simulink model "hilbert_example"  (R2024a)
settings: Solver=VariableStepAuto  StartTime=0.0  StopTime=10.0  RelTol=1e-3
model workspace (MAT data in the model file):
  ADC_BIT_RESOLUTION = 8
  ADC_BUFFER_SIZE = 1024
  ADC_Q_INTERVAL = 1
undefined symbols (not defined in the file): fdesignblkfcn, gcbh
libraries: dspxfrm3 x2
settings Model: Creator=94410  LastModifiedBy=94410

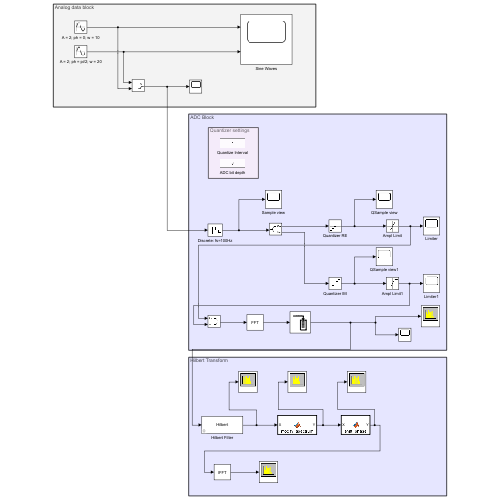
[thumbnail: Simulink's stored preview of the top-level diagram]
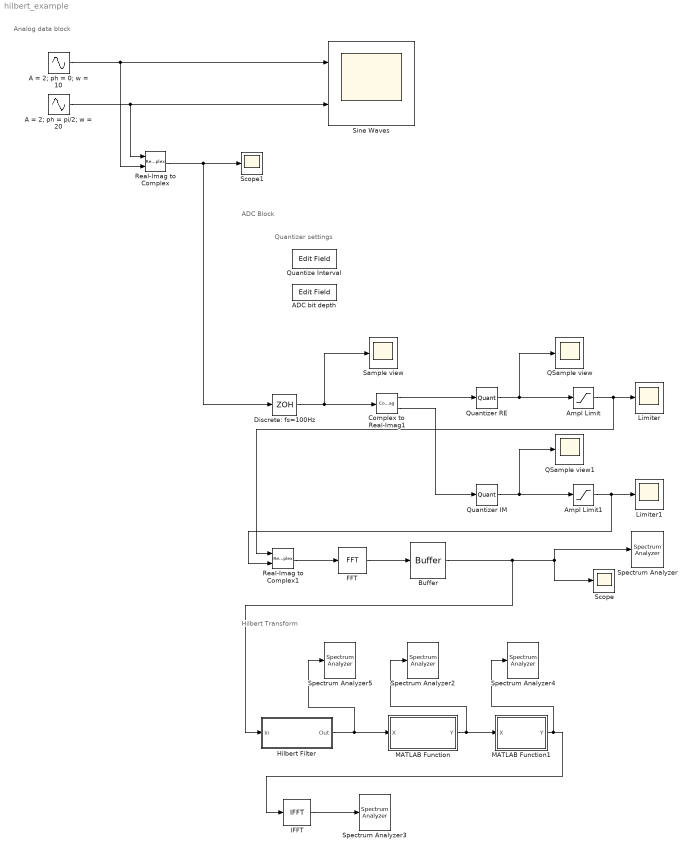
== system hilbert_example ==
  note: Hilbert Transform
  note: Quantizer settings
  note: Analog data block
  note: ADC Block
  A = 2; ph = 0; w = 10 : Sin  Amplitude=2  Frequency=10  SampleTime=0
  A = 2; ph = pi/2; w = 20 : Sin  Amplitude=2  Frequency=20  Phase=pi/2  SampleTime=0
  ADC bit depth : EditField  LabelPosition=Hide  ShowInitialText=on  Alignment=Center
  Ampl Limit : Saturate  UpperLimit=5  LowerLimit=-5
  Ampl Limit1 : Saturate  UpperLimit=5  LowerLimit=-5
  Buffer : Buffer  OutputFrames=off
  Complex to Real-Imag1 : ComplexToRealImag
  Discrete: fs=100Hz : ZeroOrderHold  SampleTime=0.01
  FFT : dspxfrm3/FFT  FFTImplementation=Auto  CompMethod=Table lookup  TableOpt=NEW  TableOptActive=Speed  BitRevOrder=off  Normalize=off  InheritFFTLength=on  FFTLength=64  WrapInput=on  roundingMode=Ceiling  overflowMode=off  firstCoeffDataTypeStr=Inherit: Same word length as input  firstCoeffLastDataTypeStr=Inherit: Same word length as input  outputMin=[]  outputMax=[]
  Hilbert Filter : Subsystem  DialogController=fdesignblkfcn  InitFcn=fdesignblkfcn(gcbh, {'InitFcn'});  mask(Hilbert Filter){}
      mask help: dsp:DSPFilterDesignBlockDialog:HilbertFdesign_MaskDesc
      settings: CopyFcn=fdesignblkfcn(gcbh, {'CopyFcn'});
      mask Help: helpview(mapfilelocation('dsp'), 'dsphilbertfilter');
      mask Display: disp('Hilbert')
  IFFT : dspxfrm3/IFFT  FFTImplementation=Auto  CompMethod=Table lookup  TableOpt=NEW  TableOptActive=Speed  BitRevOrder=off  cs_in=off  Normalize=on  InheritFFTLength=on  FFTLength=64  WrapInput=on  mode=Real  outSamplingMode=Sample based  roundingMode=Ceiling  overflowMode=off  firstCoeffDataTypeStr=Inherit: Same word length as input  firstCoeffLastDataTypeStr=Inherit: Same word length as input  outputMin=[]  outputMax=[]
  Limiter : Scope
  Limiter1 : Scope
  MATLAB Function : MATLAB Function  TreatAsAtomicUnit=on
  MATLAB Function1 : MATLAB Function  TreatAsAtomicUnit=on
  QSample view : Scope
  QSample view1 : Scope
  Quantize Interval : EditField  LabelPosition=Hide  ShowInitialText=on  Alignment=Center
  Quantizer IM : Quantizer  QuantizationInterval=ADC_Q_INTERVAL/(2^ADC_BIT_RESOLUTION)  LinearizeAsGain=off
  Quantizer RE : Quantizer  QuantizationInterval=ADC_Q_INTERVAL/(2^ADC_BIT_RESOLUTION)  LinearizeAsGain=off
  Real-Imag to Complex : RealImagToComplex
  Real-Imag to Complex1 : RealImagToComplex
  Sample view : Scope
  Scope : Scope
  Scope1 : Scope
  Sine Waves : Scope  NumInputPorts=2
  Spectrum Analyzer : SpectrumAnalyzer  WindowPosition=[355.000000,-231.000000,1318.000000,670.000000,]  ScopeFrameLocation=window  InputDomain=Frequency  Span=100  StartFrequency=-50  StopFrequency=50  InputUnits=None  SpectrumUnits=Auto  YLimits=[-2.5,2.5]  SelectedToolstripTab=spectrumAnalyzerToolstrip.channelMeasurementsTab
  Spectrum Analyzer2 : SpectrumAnalyzer  WindowPosition=[306.000000,180.000000,789.000000,436.000000,]  ScopeFrameLocation=window  InputDomain=Frequency  Span=100  StartFrequency=-50  StopFrequency=50  InputUnits=None  SpectrumUnits=Auto  YLimits=[-3.73353184,2.69746606]  SelectedToolstripTab=spectrumAnalyzerToolstrip.measurementsTab
  Spectrum Analyzer3 : SpectrumAnalyzer  WindowPosition=[266.000000,181.000000,1327.000000,750.000000,]  ScopeFrameLocation=window  InputDomain=Frequency  Span=100  StartFrequency=-50  StopFrequency=50  InputUnits=None  SpectrumUnits=Auto  YLimits=[-72.37843593,8.44661924]  SelectedToolstripTab=spectrumAnalyzerToolstrip.estimationTab
  Spectrum Analyzer4 : SpectrumAnalyzer  WindowPosition=[148.000000,72.000000,1242.000000,717.000000,]  ScopeFrameLocation=window  InputDomain=Frequency  Span=100  StartFrequency=-50  StopFrequency=50  InputUnits=None  SpectrumUnits=Auto  YLimits=[-1.91256104,2.64464345]
  Spectrum Analyzer5 : SpectrumAnalyzer  WindowPosition=[436.000000,73.000000,1242.000000,717.000000,]  ScopeFrameLocation=window  InputDomain=Frequency  Span=100  StartFrequency=-50  StopFrequency=50  InputUnits=None  SpectrumUnits=Auto  YLimits=[-61.42039238,37.54707884]  SelectedToolstripTab=spectrumAnalyzerToolstrip.measurementsTab
  wires:
  A = 2; ph = pi/2; w = 20/1 -> Real-Imag to Complex/1, Sine Waves/2
  A = 2; ph = 0; w = 10/1 -> Real-Imag to Complex/2, Sine Waves/1
  Quantizer RE/1 -> Ampl Limit/1, QSample view/1
  Ampl Limit/1 -> Real-Imag to Complex1/1, Limiter/1
  Real-Imag to Complex/1 -> Scope1/1, Discrete: fs=100Hz/1
  Discrete: fs=100Hz/1 -> Complex to Real-Imag1/1, Sample view/1
  Complex to Real-Imag1/1 -> Quantizer RE/1
  Ampl Limit1/1 -> Real-Imag to Complex1/2, Limiter1/1
  Quantizer IM/1 -> Ampl Limit1/1, QSample view1/1
  Complex to Real-Imag1/2 -> Quantizer IM/1
  Real-Imag to Complex1/1 -> FFT/1
  FFT/1 -> Buffer/1
  Buffer/1 -> Hilbert Filter/1(In), Spectrum Analyzer/1, Scope/1
  Hilbert Filter/1(Out) -> Spectrum Analyzer5/1, MATLAB Function/1(X)
  MATLAB Function/1(Y) -> Spectrum Analyzer2/1, MATLAB Function1/1(X)
  MATLAB Function1/1(Y) -> Spectrum Analyzer4/1, IFFT/1
  IFFT/1 -> Spectrum Analyzer3/1

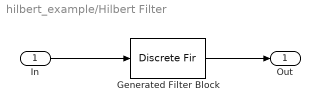
== system hilbert_example/Hilbert Filter ==
  In : Inport
  Generated Filter Block : DiscreteFir  Tag=BlockMethodSubSystem  Coefficients=[-0.026449858259791379 -0.00578355491829027 -0.016572261903348456 -0.0095390561131982743 -0.022461390535071568 -0.014999256435125952 -0.030323967074738556 -0.023012528163449009 -0.041429315821655127 -0.035762828939278346 -0.05911752381753177 -0.059034685410808696 -0.094459906652176406 -0.11739830204172252 -0.21797718993610349 -0.62869353747279177 0.62869353747279177 0.21797718993610349 0.11739830204172252 0.094459906652176406 0.059034685410808696 0.05911752381753177 0.035762828939278346 0.041429315821655127 0.023012528163449009 0.030323967074738556 0.014999256435125952 0.022461390535071568 0.0095390561131982743 0.016572261903348456 0.00578355491829027 0.026449858259791379]  InputProcessing=Columns as channels (frame based)
  Out : Outport  VectorParamsAs1DForOutWhenUnconnected=off
  wires:
  Generated Filter Block/1 -> Out/1
  In/1 -> Generated Filter Block/1

== matlab function hilbert_example/MATLAB Function ==
  data: X input; Y output
function Y = modify_spectrum(X)
    N = length(X);
    Y = X;
    Y(1:round(N/4)) = Y(1:round(N/4)) * 0.5;  % Ослабить низкие частоты
    Y(round(3*N/4):end) = Y(round(3*N/4):end) * 1.5; % Усилить высокие частоты
end

== matlab function hilbert_example/MATLAB Function1 ==
  data: X input; Y output
function Y = shift_phase(X)
    Y = X .* exp(1j * pi / 2);
end
